simulink model "Demo1_P1A2"  (R2023a)
settings: Solver=VariableStepAuto  StartTime=0.0  StopTime=20.0  RelTol=1e-3
settings Model: Creator=rqouta  LastModifiedBy=rqouta

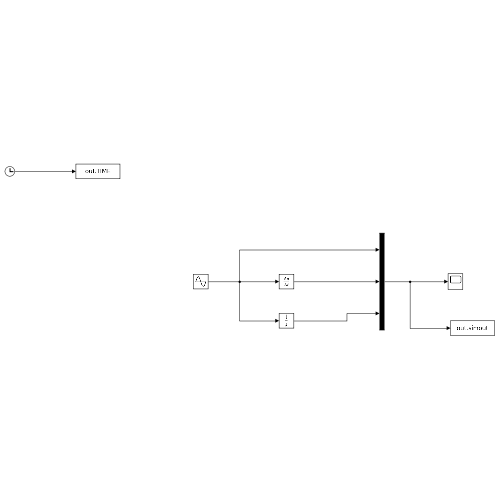
[thumbnail: Simulink's stored preview of the top-level diagram]
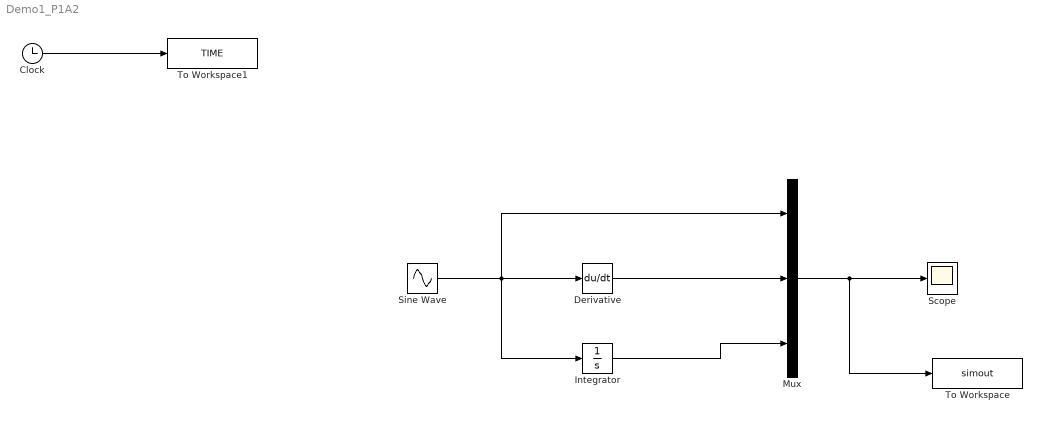
== system Demo1_P1A2 ==
  Clock : Clock
  Derivative : Derivative
  Integrator : Integrator
  Mux : Mux  Inputs=3
  Scope : Scope
  Sine Wave : Sin  Frequency=1.256  SampleTime=0
  To Workspace : ToWorkspace  VariableName=simout  SampleTime=-1
  To Workspace1 : ToWorkspace  VariableName=TIME  SampleTime=-1
  wires:
  Derivative/1 -> Mux/2
  Sine Wave/1 -> Mux/1, Integrator/1, Derivative/1
  Integrator/1 -> Mux/3
  Mux/1 -> To Workspace/1, Scope/1
  Clock/1 -> To Workspace1/1
